simulink model "test_3_31"  (R2021a)
settings: Solver=VariableStepAuto  StartTime=0.0  StopTime=0.03  RelTol=1e-3
libraries: spsSeriesRLCBranchLib x5, spsCurrentMeasurementLib x5, spsDiodeLib x4, spsGroundLib x4, spsMosfetLib x4, spsParallelRLCBranchLib x1, spsDCVoltageSourceLib x1, spspowerguiLib x1
settings Model: Creator=Dell  LastModifiedBy=Dell

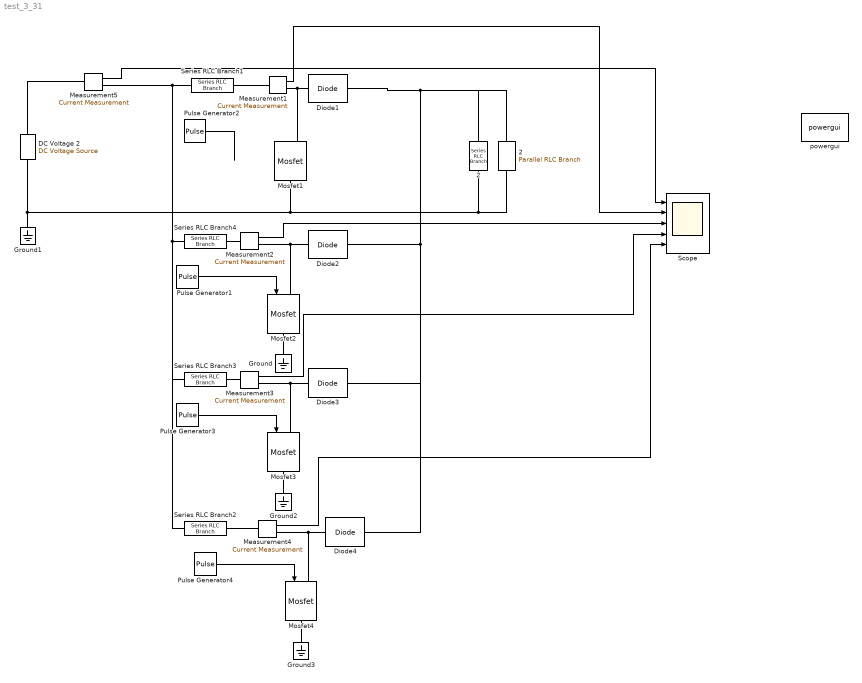
== system test_3_31 ==
  "    2" : spsSeriesRLCBranchLib/Series RLC Branch  LConnTagsString=__new0  RConnTagsString=__new0  BranchType=C  Resistance=0  Inductance=69e-3  SetiL0=off  InitialCurrent=0  Capacitance=3.2e-6  Setx0=off  InitialVoltage=0  Measurements=None
  "  2" : spsParallelRLCBranchLib/Parallel RLC Branch  LConnTagsString=a  RConnTagsString=__new0  BranchType=R  Resistance=120  Inductance=1e-3  SetiL0=off  InitialCurrent=0  Capacitance=1e-6  Setx0=off  InitialVoltage=0  Measurements=None
   Measurement{1..5} (5 alike) : spsCurrentMeasurementLib/Current Measurement  PhasorSimulation=off  OutputType=Complex  PSBequivalent=0
  DC Voltage 2 : spsDCVoltageSourceLib/DC Voltage Source  Amplitude=15  Measurements=Voltage
  Diode{1..4} (4 alike) : spsDiodeLib/Diode  Ron=0.001  Lon=0  Vf=0.8  IC=0  UseSnubber=off  Rs=inf  Cs=250e-9  Measurements=off
  Ground{,1..3} (4 alike) : spsGroundLib/Ground  LConnTagsString=a
  Mosfet{1..4} (4 alike) : spsMosfetLib/Mosfet  Ron=0.1  Lon=0  Rd=0.01  Vfd=0  IC=0  Rs=1e5  Cs=inf  Measurements=off
  Pulse Generator1 : DiscretePulseGenerator  PulseType=Time based  Period=1/100000  PulseWidth=60  PhaseDelay=1/400000
  Pulse Generator2 : DiscretePulseGenerator  PulseType=Time based  Period=1/100000  PulseWidth=60
  Pulse Generator3 : DiscretePulseGenerator  PulseType=Time based  Period=1/100000  PulseWidth=60  PhaseDelay=2/400000
  Pulse Generator4 : DiscretePulseGenerator  PulseType=Time based  Period=1/100000  PulseWidth=60  PhaseDelay=3/400000
  Scope : Scope  NumInputPorts=5
  Series RLC Branch{1..4} (4 alike) : spsSeriesRLCBranchLib/Series RLC Branch  LConnTagsString=__new0  RConnTagsString=__new0  BranchType=L  Resistance=0  Inductance=2.332e-3  SetiL0=off  InitialCurrent=0  Capacitance=1e-6  Setx0=off  InitialVoltage=0  Measurements=None
  powergui : spspowerguiLib/powergui  Priority=1  SimulationMode=Discrete  SampleTime=2.5e-8  frequency=60  Iterations=50  frequencyindice=0  Pbase=100e6  ErrMax=1e-4  UnitsV=kV  UnitsW=MW  buscounter=0  FunctionMessages=off  echomessages=off  EnableUseOfTLC=off  CurrentSourceSwitches=on  DisableSnubberDevices=off  DisableRonSwitches=off  DisableVfSwitches=off  DisplayEquations=off  AutomaticDiscreteSolvers=off  SolverType=Tustin  Interpol=off  ExternalGateDelay=off  methode=off  Ts=100  x0status=blocks  SPID=off  SwTol=0  HookPort=off  NonlinearTolerance=1e-4  nMaxIteration=100  ContinueOnMaxIteration=off  RestoreLinks=warning  ResistiveCurrentMeasurement=off  Frange=[0:2:500]  Ylog=off  Xlog=on  ShowGrid=off  save=off  variable=ZData  structure=ScopeData  ZoomFFT=off  StartTime=0.033333  cycles=1  DisplayStyle=1  fundamental=300000  FreqAxis=on  MaxFrequency=300000  frequencyindicesteady=1  RmsSteady=1  display=off
  wires:
  Pulse Generator2/1 -> ?
  Pulse Generator1/1 -> Mosfet2/1
  " Measurement1"/1 -> Scope/2
  " Measurement2"/1 -> Scope/3
  Pulse Generator3/1 -> Mosfet3/1
  " Measurement3"/1 -> Scope/4
  Pulse Generator4/1 -> Mosfet4/1
  " Measurement4"/1 -> Scope/5
  " Measurement5"/1 -> Scope/1
  connections:
  " Measurement1"/RConn1 -- Mosfet1/LConn1 -- Diode1/LConn1
  "    2"/RConn1 -- Mosfet1/RConn1 -- DC Voltage 2/LConn1 -- Ground1/LConn1 -- "  2"/RConn1
  Diode1/RConn1 -- "  2"/LConn1 -- "    2"/LConn1 -- Diode4/RConn1 -- Diode3/RConn1 -- Diode2/RConn1
  " Measurement1"/LConn1 -- Series RLC Branch1/RConn1
  Series RLC Branch4/LConn1 -- Series RLC Branch3/LConn1 -- Series RLC Branch2/LConn1 -- Series RLC Branch1/LConn1 -- " Measurement5"/RConn1
  Ground/LConn1 -- Mosfet2/RConn1
  Diode2/LConn1 -- " Measurement2"/RConn1 -- Mosfet2/LConn1
  " Measurement2"/LConn1 -- Series RLC Branch4/RConn1
  Diode3/LConn1 -- " Measurement3"/RConn1 -- Mosfet3/LConn1
  Series RLC Branch3/RConn1 -- " Measurement3"/LConn1
  Ground2/LConn1 -- Mosfet3/RConn1
  Diode4/LConn1 -- " Measurement4"/RConn1 -- Mosfet4/LConn1
  " Measurement4"/LConn1 -- Series RLC Branch2/RConn1
  Ground3/LConn1 -- Mosfet4/RConn1
  " Measurement5"/LConn1 -- DC Voltage 2/RConn1
